simulink model "Feedback_Effect"  (R2024b)
settings: Solver=FixedStepAuto  StartTime=0.0  StopTime=10.0  FixedStep=0.001  RelTol=1e-3
settings Model: Creator=abdal  LastModifiedBy=abdal

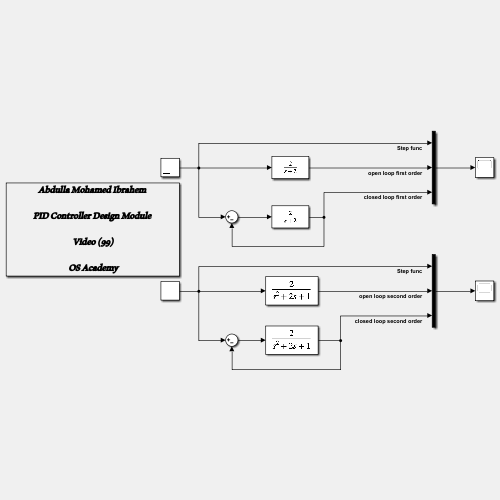
[thumbnail: Simulink's stored preview of the top-level diagram]
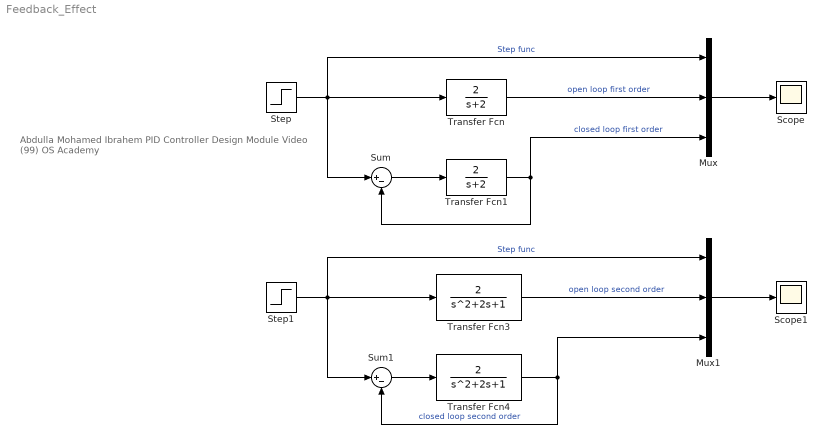
== system Feedback_Effect ==
  note: Abdulla Mohamed Ibrahem
      | PID Controller Design Module
      | Video (99)
      | OS Academy
  Mux : Mux  Inputs=3
  Mux1 : Mux  Inputs=3
  Scope : Scope
  Scope1 : Scope
  Step : Step  SampleTime=0
  Step1 : Step  SampleTime=0
  Sum : Sum  Inputs=|+-
  Sum1 : Sum  Inputs=|+-
  Transfer Fcn : TransferFcn  Numerator=[2]  Denominator=[1 2]
  Transfer Fcn1 : TransferFcn  Numerator=[2]  Denominator=[1 2]
  Transfer Fcn3 : TransferFcn  Numerator=[2]
  Transfer Fcn4 : TransferFcn  Numerator=[2]
  wires:
  Step/1 -> Mux/1, Transfer Fcn/1, Sum/1  "Step func"
  Transfer Fcn1/1 -> Mux/3, Sum/2  "closed loop first order"
  Transfer Fcn/1 -> Mux/2  "open loop first order"
  Mux/1 -> Scope/1
  Sum/1 -> Transfer Fcn1/1
  Sum1/1 -> Transfer Fcn4/1
  Mux1/1 -> Scope1/1
  Transfer Fcn3/1 -> Mux1/2  "open loop second order"
  Transfer Fcn4/1 -> Sum1/2, Mux1/3  "closed loop second order"
  Step1/1 -> Sum1/1, Transfer Fcn3/1, Mux1/1  "Step func"
